simulink model "Parallel3"  (Simulink 5.0)
settings: Solver=ode45  StartTime=0.0  StopTime=10.0  RelTol=1e-3
settings Model: Creator=scaife  LastModifiedBy=scaife  ExtModeAutoUpdateStatusClock=off

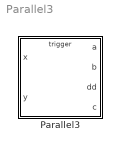
== system Parallel3 ==
  Parallel3 : Stateflow chart

== stateflow chart Parallel3 ==
  state A [parallel]
    state A1
      state A1a/
        en:a=x+1
      state A1b/
        en:a=x+2
      A1a -> A1b : S
      A1b -> A1a : R
      (default) -> A1a
    state A2
      state A2a/
        en:a=x+3
      state A2b/
        en:a=x+4
      (default) -> A2a
      A2a -> A2b : S
      A2b -> A2a : R
    A1 -> A2 : T
    A2 -> A1 : T
    (default) -> A1
  state B [parallel]
    state B2
      state B2a/
        en:b=x+7
      state B2b/
        en:b=x+8
      (default) -> B2a
      B2b -> B2a : R
      B2a -> B2b : S
    state B1
      state B1a/
        en:b=x+5
      state B1b/
        en:b=x+6
      (default) -> B1a
      B1a -> B1b : S
      B1b -> B1a : R
    (default) -> B1
    B1 -> B2 : T
    B2 -> B1 : T
  state C [parallel]
    state C2
      state C2a/
        en:c=y+3
      state C2b/
        en:c=y+4
      (default) -> C2a
      C2b -> C2a : R
      C2a -> C2b : S
    state C1
      state C1a/
        en:c=y+1
      state C1b/
        en:c=y+2
      (default) -> C1a
      C1b -> C1a : R
      C1a -> C1b : S
    (default) -> C1
    C1 -> C2 : T
    C2 -> C1 : T
  state D [parallel]
    state D2
      state D2a/
        en:dd=y+7
      state D2b/
        en:dd=y+8
      (default) -> D2a
      D2a -> D2b : S
      D2b -> D2a : R
    state D1
      state D1a/
        en:dd=y+5
      state D1b/
        en:dd=y+6
      (default) -> D1a
      D1a -> D1b : S
      D1b -> D1a : R
    (default) -> D1
    D1 -> D2 : T
    D2 -> D1 : T
  data: a output int32; b output int32; dd output int32; c output int32; x input int32; y input int32
  events: R input EITHER_EDGE_EVENT; S input EITHER_EDGE_EVENT; T input EITHER_EDGE_EVENT
